simulink model "test_com_SensorFusion_SF_E10_fuerE9Daten"  (R2019b)
settings: Solver=FixedStepDiscrete  StartTime=0  StopTime=85  FixedStep=0.001  RelTol=1e-3
undefined symbols (not defined in the file or in its folder): BxTM, ByTM, CxTM, CyTM, g, gamma_stat_front, gamma_stat_rear, gearbox_ratio, l_F, l_R, m_sprung, m_unsprung_quarter, mag_calib_front_center, mag_calib_front_compmatrix, mag_calib_rear_center, mag_calib_rear_compmatrix, param, switch_VelYcalculation_pSF, testStart_VelX_pSF, testVelY_pSF, tire_r_dyn, track_angle_front, track_width_front, track_width_rear, v2o_x, wheel_kinematics_breakpoints, wheel_kinematics_FL_data, wheel_kinematics_FR_data, wheelbase, x9DFrontX, x9DFrontY, x9DRearX, x9DRearY
libraries: SignalProcessingSensorFusionLib x30, simulink x3
(part 5 of 7)

== matlab function test_com_SensorFusion_SF_E10_fuerE9Daten/Subsystem14/simple_TireLoadEstimation/MATLAB Function ==
  data: a_x input; F_z_vl output; a_y input; F_z_vr output; F_z_hl output; F_z_hr output
function [F_z_vl, F_z_vr, F_z_hl, F_z_hr] = Radlast_Beschleunigung_e9_SAE(a_x, a_y)
m=240;
g=9.81;
l=1.540;
l_v=0.796;
l_h=l-l_v;
h_s=0.2648;
b_v=0.6*2;
b_h=0.6*2;
F_z_vl=single(0);
F_z_vr=single(0);
F_z_hl=single(0);
F_z_hr=single(0);
 %m=Fahrzeugmasse; h_s= Schwerpunktshöhe (von SP zu Anbindung von Rods an Radträger); l_h= Abstand von HA zu
 %SP; l_v=Radstand von VA zum SP l=Radstand; a_x=Beschleunigung in x-Richtung; a_y=Beschleunigung
 %in y-Richtung; b_v=Spurbreite vorne;b_h=Spurbreite hinten; 
 
 %EDITIERT, so dass Vorzeichen vor h_s*a_y/(b_v*g) jeweils getauscht wurde

m_ges_f= m * (l-l_v)/l;
m_ges_r= m * l_v/l;
Delta_TireLoad_x = m * (h_s/(2*l))*a_x; %die 2 hier ist in E7 Radlastschätzer nicht so drin
%{ TireLoad = [...
%    m_ges_f *(0.5*g + (h_s/b_v)* a_y) - Delta_TireLoad_x ...
%    m_ges_f *(0.5*g - (h_s/b_v)* a_y) - Delta_TireLoad_x ...
%    m_ges_r *(0.5*g + (h_s/b_h)* a_y) + Delta_TireLoad_x ...
%    m_ges_r *(0.5*g - (h_s/b_h)* a_y) + Delta_TireLoad_x];
%}

TireLoad = [ ...
    m*(l_h*g-h_s*a_x)*(0.5+(h_s*a_y/(b_v*g)))/l;
    m*(l_h*g-h_s*a_x)*(0.5-(h_s*a_y/(b_v*g)))/l;
    m*(l_v*g+h_s*a_x)*(0.5+(h_s*a_y/(b_h*g)))/l;
    m*(l_v*g+h_s*a_x)*(0.5-(h_s*a_y/(b_h*g)))/l
    ];
if TireLoad(1)<0
    F_z_vl = single(0);
else
    F_z_vl = TireLoad(1);
end

if TireLoad(2)<0
    F_z_vr = single(0);
else
    F_z_vr = TireLoad(2);
end

if TireLoad(3)<0
    F_z_hl = single(0);
else
    F_z_hl = TireLoad(3);
end

if TireLoad(4)<0
    F_z_hr = single(0);
else
    F_z_hr = TireLoad(4);
end

end

== matlab function test_com_SensorFusion_SF_E10_fuerE9Daten/Subsystem14/SensorFusion_E8_adjusted/SensorFusion/kalman ==
  data: x9DFront input; x9DRear input; VehicleState output Bus: control_VehicleState size=1; bias output single size=6; Heading output single size=[2 1]; Covariance output single size=[13,13]; v2o input; WheelSpeeds input; rockerAngles input; wheelTorques input; wheelAngles input; driverInputs input; x9DFrontX parameter; x9DFrontY parameter; x9DRearX parameter; x9DRearY parameter; v2o_x parameter; mag_calib_front_center parameter; mag_calib_front_compmatrix parameter; mag_calib_rear_center parameter; mag_calib_rear_compmatrix parameter; track_width_front parameter; track_width_rear parameter; z_out output Bus: debug_measurementsAtCOG
function [VehicleState, bias, Heading, Covariance, z_out] = fcn(x9DFront, x9DRear, v2o, WheelSpeeds, rockerAngles, wheelTorques, wheelAngles, driverInputs, x9DFrontX,x9DFrontY, x9DRearX, x9DRearY, v2o_x, mag_calib_front_center, mag_calib_front_compmatrix, mag_calib_rear_center, mag_calib_rear_compmatrix, track_width_front, track_width_rear)

persistent x P k Heading_Rear_old Heading_Front_old testsumme magnetoffset i testsumme2 testsumme3 v2o_VelX_old

%% Setup

% kalman filter
% x_k+1 = F x_k + w_k
% z_k = H x_k + v_k

% State vector
% x = [a_x_c;     % (1)   Acceleration in x-direction of the car (CG)
%      a_y_c;     % (2)        -"-        y-direction  
%      v_x_c;     % (3)   Velocity in x-direction
%      v_y_c;     % (4)        -"-    y-direction
%      psi_c;     % (5)   Yaw angle of the car
%      r_c;       % (6)   Yaw rate     -"-
%      r_d_c;     % (7)   Yaw acceleration
%      b_x_a1;    % (8)   Bias 1. acceleration sensor in x-direction
%      b_y_a1;    % (9)                -"-               y-direction
%      b_x_a2;    % (10)  Bias 2. acceleration sensor in x-direction
%      b_y_a2;    % (11)               -"-               y-direction
%      b_r1;      % (12)  Bias 1. gyroscope around z-axis
%      b_r2];     % (13)  Bias 2.          -"-
% 

% sample time dt [seconds]
num_states=13;
dt=0.002;

Heading = single(zeros(2,1));

if isempty(P)
%init

% Transformation  (normative matrix * (measured signal - offset))
CompCorrFront = mag_calib_front_compmatrix * ([x9DFront.MagX; x9DFront.MagY; x9DFront.MagZ] - mag_calib_front_center);
CompCorrRear = mag_calib_rear_compmatrix * ([x9DRear.MagX; x9DRear.MagY; x9DRear.MagZ] - mag_calib_rear_center);

% Yaw angle calculation based on normalized magnetic compass data

Heading_Front_old = -1*atan2(CompCorrFront(2,:), CompCorrFront(1,:)); % intervall [0,2*pi];
Heading_Rear_old = -1*atan2(CompCorrRear(2,:), CompCorrRear(1,:)); % intervall [0,2*pi];

Heading_Front_old = -Heading_Front_old;
Heading_Rear_old = -Heading_Rear_old;

i=1;
% testsumme = zeros(1,24);
% testsumme2 = zeros(1,24);
% testsumme3 = zeros(1,24);

magnetoffset = Heading_Rear_old - Heading_Front_old;

state = 0;

v2o_VelX_old=single(0);
k = 1;
x = single(zeros(num_states,1));
x(5) = Heading_Front_old;
P = single(zeros(num_states, num_states));

Heading_Front_old = Heading_Front_old + magnetoffset; % intervall [0,2*pi];


end

%% Transformation of measured signals

% Transformation  (normative matrix * (measured signal - offset))
CompCorrFront = mag_calib_front_compmatrix * ([x9DFront.MagX; x9DFront.MagY; x9DFront.MagZ] - mag_calib_front_center);
CompCorrRear = mag_calib_rear_compmatrix * ([x9DRear.MagX; x9DRear.MagY; x9DRear.MagZ] - mag_calib_rear_center);

% Yaw angle calculation based on normalized magnetic compass data


HeadingFront = -1*atan2(CompCorrFront(2,:), CompCorrFront(1,:)) + magnetoffset; % intervall [0,2*pi];
HeadingRear = -1*atan2(CompCorrRear(2,:), CompCorrRear(1,:)); % intervall [0,2*pi];


HeadingFront = -HeadingFront;
HeadingRear = -HeadingRear;

if(Heading_Front_old-HeadingFront < -pi)
HeadingFront = HeadingFront - round(abs(Heading_Front_old-HeadingFront)/(2*pi))*2*pi;
elseif(Heading_Front_old-HeadingFront > pi)
HeadingFront = HeadingFront + round(abs(Heading_Front_old-HeadingFront)/(2*pi))*2*pi;
end

if(Heading_Rear_old-HeadingRear < -pi)
HeadingRear = HeadingRear - round(abs(Heading_Rear_old-HeadingRear)/(2*pi))*2*pi;
elseif(Heading_Rear_old-HeadingRear > pi)
HeadingRear = HeadingRear + round(abs(Heading_Rear_old-HeadingRear)/(2*pi))*2*pi;
end


Heading_Front_old = HeadingFront;
Heading_Rear_old = HeadingRear;

% Korrektur des Gyroskopsensors mit Temperaturdaten

r_m1 = x9DFront.YawRate - 1.3 * 0 * x9DFront.Temperature;       % TODO: Anpassen an tatsächliche Sensoren und auslagern als Parameter
r_m2 = x9DRear.YawRate - 1.3 * 0 * x9DRear.Temperature;

%% Plausibilisierung der Sensorwerte

% Differenz durchschnittl. Raddrehzahl / Schwimmwinkelsensor > Schwellwert
% -> Schwimmwinkelsensor nicht vertrauen

WheelSpeeds(1) = WheelSpeeds(1) * 0.221; % dynamischer Reifenradius
WheelSpeeds(2) = WheelSpeeds(2) * 0.221; % dynamischer Reifenradius
WheelSpeeds(3) = WheelSpeeds(3) * 0.221; % dynamischer Reifenradius
WheelSpeeds(4) = WheelSpeeds(4) * 0.221; % dynamischer Reifenradius

% Durchschnittliche Raddrehzahl ermitteln
avgWheelSpeed = ( WheelSpeeds(1) + WheelSpeeds(2) +...
    WheelSpeeds(3) + WheelSpeeds(4) ) / 4;

% Raddrehzahlen in Vektor speichern um minimale/maximale Raddrehzahl
% bestimmen zu können
WheelSpeedsVec = [WheelSpeeds(1), WheelSpeeds(2), ...
    WheelSpeeds(3), WheelSpeeds(4)];
WheelDistances = [-track_width_front/2, track_width_front/2, ...
    -track_width_rear/2, track_width_rear/2];

% Wenn Längsbeschleunigung positiv, minimale Raddrehzahl benutzen. Wenn
% negativ maximale Raddrehzahl benutzen..
if x(1) > 0
[MinWheelSpeed,index] = min(WheelSpeedsVec);
MinWheelDistY = WheelDistances(index);
else
    [MinWheelSpeed,index] = max(WheelSpeedsVec);
     MinWheelDistY = WheelDistances(index);
end

%% valueIsNew Slipangle Sensor
valueIsNew = false;
if(v2o_VelX_old~=single(v2o.VelX))
    valueIsNew = true;
    v2o_VelX_old=single(v2o.VelX);
end

%% Prediction

% System matrix
F =[
    [ 0, 0, 0, 0, 0, 0, 0, 0, 0, 0, 0, 0, 0]
    [ 0, 0, 0, 0, 0, 0, 0, 0, 0, 0, 0, 0, 0]
    [ 1, 0, 0, 0, 0, 0, 0, 0, 0, 0, 0, 0, 0]
    [ 0, 1, 0, 0, 0, 0, 0, 0, 0, 0, 0, 0, 0]
    [ 0, 0, 0, 0, 0, 1, 0, 0, 0, 0, 0, 0, 0]
    [ 0, 0, 0, 0, 0, 0, 1, 0, 0, 0, 0, 0, 0]
    [ 0, 0, 0, 0, 0, 0, 0, 0, 0, 0, 0, 0, 0]
    [ 0, 0, 0, 0, 0, 0, 0, 0, 0, 0, 0, 0, 0]
    [ 0, 0, 0, 0, 0, 0, 0, 0, 0, 0, 0, 0, 0]
    [ 0, 0, 0, 0, 0, 0, 0, 0, 0, 0, 0, 0, 0]
    [ 0, 0, 0, 0, 0, 0, 0, 0, 0, 0, 0, 0, 0]
    [ 0, 0, 0, 0, 0, 0, 0, 0, 0, 0, 0, 0, 0]
    [ 0, 0, 0, 0, 0, 0, 0, 0, 0, 0, 0, 0, 0]
   ];

A = dt*F + eye(length(F));

W = eye(num_states);
 

% Covariance matrix of state noise
Q = diag([0.001;                        % (1)   Acceleration in x-direction of the car (CG)
          0.001;                         % (2)        -"-        y-direction  
          0.001;                         % (3)   Velocity in x-direction
          0.001;                         % (4)        -"-    y-direction
          0.01;                         % (5)   Yaw angle of the car
          0.0001;                         % (6)   Yaw rate     -"-
          0.001;                         % (7)   Yaw acceleration
          0.1e-6;                        % (8)   Bias 1. acceleration sensor in x-direction
          0.1e-6;                         % (9)                -"-               y-direction
          0.1e-6;                        % (10)  Bias 2. acceleration sensor in x-direction
          0.1e-6;                         % (11)               -"-               y-direction
          0.1e-6;                     % (12)  Bias 1. gyroscope around z-axis
          0.1e-6]*0.002);             % (12)  Bias 2.      -"-
      
% prediction calculation
x = x + dt*F*x; % + dt*B*u;          % statevector update
P = A*P*A' + W*Q*W';                 % covariance matrix update

% testsumme(12:24) = testsumme(12:24) + dt*F(4,:).*x';
% testsumme2(12:24) = testsumme2(12:24) + dt*F(13,:).*x';
% testsumme3(12:24) = testsumme3(12:24) + dt*F(6,:).*x';

%% Correction

% Measurement equation
h = [
     x(1) + x(8);                       % (1)   x-Acc (front)
     x(2) + x(9);                       % (2)   y-Acc (front)
     x(1) + x(10);                      % (3)   x-Acc (rear)
     x(2) + x(11);                      % (4)   y-Acc (rear)
     x(6) + x(12);                      % (5)   yaw-rate (front)
     x(6) + x(13);                      % (6)   yaw-rate (rear)
     x(3); % - x(6)*v2oY*0;             % (7)   x-velocity
     x(4);                              % (8)   y-velocity
     x(5);                              % (9)   yaw-angle (front)
     x(5);                              % (10)  yaw-angle (rear)
     x(7);                              % (11)  yaw-acceleration
     x(3);                              % (12)  wheelspeed of slowes/fastest wheel (acceleration/braking)
     x(1);
     x(2);
     x(3);
     x(4);
     x(6)
     ];

% Measured states
z = [
     x9DFront.AccX - x(6)^2*x9DFrontX;                                         % (1)   x-Acc (front)
     x9DFront.AccY + x(7)*x9DFrontX;                                         % (2)   y-Acc (front)
     x9DRear.AccX - x(6)^2*x9DRearX ;                                          % (3)   x-Acc (rear)
     x9DRear.AccY + x(7)*x9DRearX;                                          % (4)   y-Acc (rear)
     r_m1;                                                  % (5)   yaw-rate (front)
     r_m2;                                                  % (6)   yaw-rate (rear)
     v2o.VelX;                              % (7)   x-velocity
     v2o.VelY + x(6)*v2o_x;                                   % (8)   y-velocity
     HeadingFront;                                          % (9)   yaw-angle (front)
     HeadingRear;                                           % (10)  yaw-angle (rear)
     x9DFront.AccY/x9DFrontX + x9DRear.AccY/x9DRearX  - (x(9)/x9DFrontX + x(11)/x9DRearX);        % (11)  yaw-acceleration
     MinWheelSpeed  + MinWheelDistY * x(6);
     0;
     0;
     0;
     0;
     0
     ];

% Jacobian of measurement equation
H =[ 
    [ 1, 0, 0, 0, 0, 2*x9DFrontX*x(6)*0,            0, 1,             0, 0,             0, 0, 0]
    [ 0, 1, 0, 0, 0,                  0, -x9DFrontX*0, 0,             1, 0,             0, 0, 0]
    [ 1, 0, 0, 0, 0,  2*x9DRearX*x(6)*0,            0, 0,             0, 1,             0, 0, 0]
    [ 0, 1, 0, 0, 0,                  0,  -x9DRearX*0, 0,             0, 0,             1, 0, 0]
    [ 0, 0, 0, 0, 0,                  1,            0, 0,             0, 0,             0, 1, 0]
    [ 0, 0, 0, 0, 0,                  1,            0, 0,             0, 0,             0, 0, 1]
    [ 0, 0, 1, 0, 0,                  0,            0, 0,             0, 0,             0, 0, 0]
    [ 0, 0, 0, 1, 0,             v2o_x*0,            0, 0,             0, 0,             0, 0, 0]
    [ 0, 0, 0, 0, 1,                  0,            0, 0,             0, 0,             0, 0, 0]
    [ 0, 0, 0, 0, 1,                  0,            0, 0,             0, 0,             0, 0, 0]
    [ 0, 0, 0, 0, 0,                  0,            1, 0, 1/x9DFrontX*0, 0,  1/x9DRearX*0, 0, 0]
    [ 0, 0, 1, 0, 0,                  0,            0, 0,             0, 0,             0, 0, 0]
    [ 1, 0, 0, 0, 0,                  0,            0, 0,             0, 0,             0, 0, 0]
    [ 0, 1, 0, 0, 0,                  0,            0, 0,             0, 0,             0, 0, 0]
    [ 0, 0, 1, 0, 0,                  0,            0, 0,             0, 0,             0, 0, 0]
    [ 0, 0, 0, 1, 0,                  0,            0, 0,             0, 0,             0, 0, 0]
    [ 0, 0, 0, 0, 0,                  1,            0, 0,             0, 0,             0, 0, 0]
   ];

R = [
     0.01;                      % (1)   x-Acc (front)
     0.01;                      % (2)   y-Acc (front)
     0.01;                      % (3)   x-Acc (rear)
     0.01;                      % (4)   y-Acc (rear)
     0.00001;                   % (5)   yaw-rate (front)
     0.00001;                   % (6)   yaw-rate (rear)
     0.0001;                    % (7)   x-velocity
     0.000001;                  % (8)   y-velocity
     0.00001;                   % (9)   yaw-angle (front)
     100.0;                     % (10)  yaw-angle (rear)
     0.001;                     % (11)  yaw-acceleration
     0.001;                     % (12)  speed of slowest wheel
     1e-20;                     % (13)  x-Acc (standstill)
     1e-20;                     % (14)  y-Acc (standstill)
     1e-20;                     % (15)  x-Vel (standstill)
     1e-20;                     % (16)  y-Vel (standstill)
     1e-20                      % (17)  Yaw-Rate (standstill)
     ];

%% Measurement selection

% Alle 4 Zeitschritte nutze Schwimmwinkeldaten -> mod(k,4)==0

if valueIsNew && abs(v2o.VelX-v2o_VelX_old) < 2 ...
        && ~xor(v2o.VelX >= 0.1 , avgWheelSpeed > 0.1)
    % Measurement equations including the v2o sensor are used if:
    %
    % - mod(k,4) because velocity is only measured every 8 ms
    %
    % - change in velocity is below 2 m/s (assumption is that a
    %   higher difference only occurs when the sensor fails)
    %
    % - ~xor(...) meaning, if v2o does show 0 and avgWheelspeed is below
    %   0.1 or if v2o doesn't show 0 and avgWheelspeed is above 0.1
    
    if (x9DFront.AccX_Sq<4)
        if (x9DRear.AccX_Sq<4)
            state = 8;
            selection = 1:11;
        else
            state = 4;
            selection = [1:2,5,7:9,12];
        end
    else
        if (x9DRear.AccX_Sq<4)
            state = 5;
            selection = [3:4,6:8,10,12];
        else
            state = 1;
            selection = 7:8;
        end    
    end
    
else
    if (x9DFront.AccX_Sq<4)
        if (x9DRear.AccX_Sq<4)
            if (v2o.VelX_Sq<4)
                state = 7;
                selection = [1:6,9:11];
            else
                state = 6;
                selection = [1:6,9:12];
            end            
        else
            state = 2;
            selection = [1,2,5,9,12];
        end
    else
        if (x9DRear.AccX_Sq<4)
            state = 3;
            selection = [3,4,6,10,12];
        else
            state = 0;
            selection = 12;
        end
    end
end

if(avgWheelSpeed < 0.1)
    selection = [selection 13:17];
end 

% 1 only slip angle sensor (slip angle)
% 2 only front 9D sensor (9D sensor)
% 3 only rear 9D sensor (9D sensor)
% 4 one 9D sensor missing (slip angle + (front) 9D sensor)
% 5 one 9D sensor missing (slip angle + (rear) 9D sensor)
% 6 long time no slip angle sensor (use motor revs for speed measurement)
% 7 no slip angle sensor (2 * 9D sensor)
% 8 all sensors available(slip angle + 2 * 9D sensors)
% 0 no sensors except wheeel speeds

%%

% (1)   x-Acc (front)
% (2)   y-Acc (front)
% (3)   x-Acc (rear)
% (4)   y-Acc (rear)
% (5)   yaw-rate (front)
% (6)   yaw-rate (rear)
% (7)   x-velocity
% (8)   y-velocity
% (9)   yaw-angle (front)
% (10)  yaw-angle (rear)
% (11)  yaw-acceleration
% (12)  wheelspeed of slowes/fastest wheel (acceleration/braking) 
% (13)  x-Acc (standstill)
% (14)  y-Acc (standstill)
% (15)  x-Vel (standstill)
% (16)  y-Vel (standstill)
% (17)  Yaw-Rate (standstill)


h_tmp = h(selection,:);
z_tmp = z(selection,:);
H_tmp = H(selection,:);
R_tmp = diag(R(selection,:));

% Correction equations
I = eye(length(x));
V_tmp = eye(length(h_tmp));

K_tmp = P*H_tmp'/(H_tmp*P*H_tmp'+V_tmp*R_tmp*V_tmp');

x = x + K_tmp*(z_tmp-h_tmp);
P = (I - K_tmp*H_tmp)*P;

%% Output 
VehicleState.PosX = single(0);
VehicleState.PosY = single(0);

VehicleState.VelX = x(3);
VehicleState.VelY = x(4);
VehicleState.YawAngle = x(5);
VehicleState.YawRate = x(6);
VehicleState.YawAcc = x(7);
VehicleState.AccX = x(1);
VehicleState.AccY = x(2);

VehicleState.AccZ = single(0);

Heading(1) = single(HeadingFront);
Heading(2) = single(HeadingRear);

z_out.AccXFront = z(1);
z_out.AccYFront = z(2);
z_out.AccXRear = z(3);
z_out.AccYRear = z(4);
z_out.YawRateFront = z(5);
z_out.YawRateRear = z(6);
z_out.VelX = z(7);
z_out.VelY = z(8);
z_out.YawAngleFront = z(9);
z_out.YawAngleRear = z(10);
z_out.YawAcceleration = z(11);


bias=x(8:13);
Covariance = P;

k = k+1;

if(i==1000)
%     
%     testsumme;
%     testsumme2;
%     testsumme3;
i = 1;
end
i = i+1;
end
